simulink model "stopwatch_extended"  (Simulink 10.1)
settings: Solver=FixedStepAuto  StartTime=0.0  StopTime=1000.0  FixedStep=1e-3  RelTol=1e-3
settings Model: Creator=Robin Vogt  LastModifiedBy=Robin Vogt  EnablePacing=on
settings DataIOCC: SaveFormat=Dataset  ReturnWorkspaceOutputs=on
settings OptimizationCC: LifeSpan=auto
settings DebuggingCC: UnderspecifiedInitializationDetection=Simplified  MergeDetectMultiDrivingBlocksExec=error  SFUnexpectedBacktrackingDiag=error  SFNoUnconditionalDefaultTransitionDiag=error  SFExecutionAtInitializationDiag=warning  ArithmeticOperatorsInVariantConditions=error
settings HardwareCC: ProdBitPerPointer=64  ProdBitPerSizeT=64  ProdBitPerPtrDiffT=64  ProdLargestAtomicFloat=Float  ProdIntDivRoundTo=Zero  ProdEndianess=LittleEndian  ProdWordSize=64  ProdHWDeviceType=Intel->x86-64 (Windows64)
settings ModelReferenceCC: PropagateSignalLabelsOutOfModel=on
settings SFSimCC: SimUseLocalCustomCode=on  CustomCodeUndefinedFunction=FilterOut
settings RTWCC: RTWUseLocalCustomCode=on
settings CodeAppCC: StateflowObjectComments=off
settings GRTTargetCC: TargetLangStandard=C99 (ISO)  CombineOutputUpdateFcns=on  GRTInterface=off
settings ConfigComp: CovMetricSettings=dwe  CovHtmlReporting=off  CovSaveCumulativeToWorkspaceVar=off  CovSaveSingleToWorkspaceVar=off  CovExternalEMLEnable=on

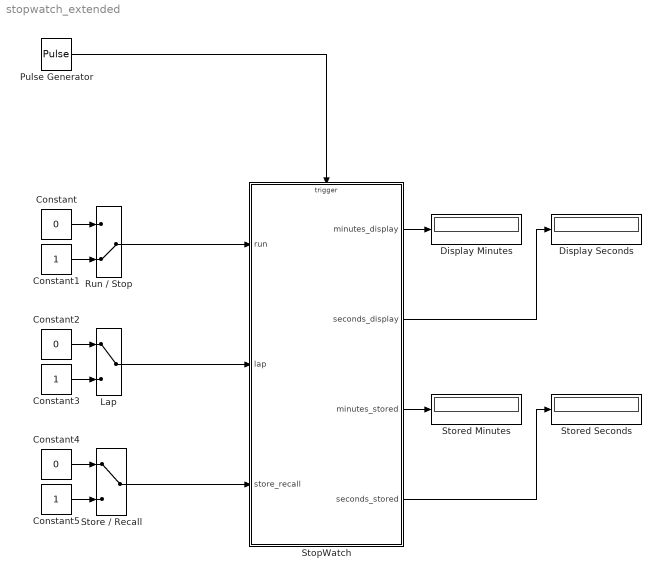
== system stopwatch_extended ==
  Constant : Constant  Value=0  OutDataTypeStr=boolean
  Constant1 : Constant  OutDataTypeStr=boolean
  Constant2 : Constant  Value=0  OutDataTypeStr=boolean
  Constant3 : Constant  OutDataTypeStr=boolean
  Constant4 : Constant  Value=0  OutDataTypeStr=boolean
  Constant5 : Constant  OutDataTypeStr=boolean
  Display Minutes : Display
  Display Seconds : Display
  Lap : ManualSwitch
  Pulse Generator : DiscretePulseGenerator  PulseType=Time based  Period=1  PulseWidth=5
  Run / Stop : ManualSwitch  CurrentSetting=0
  StopWatch : Stateflow chart  TreatAsAtomicUnit=on
  Store / Recall : ManualSwitch
  Stored Minutes : Display
  Stored Seconds : Display
  wires:
  Constant/1 -> Run / Stop/1
  Constant1/1 -> Run / Stop/2
  Run / Stop/1 -> StopWatch/1(run)
  Constant3/1 -> Lap/2
  Constant2/1 -> Lap/1
  StopWatch/2(seconds_display) -> Display Seconds/1
  StopWatch/1(minutes_display) -> Display Minutes/1
  Constant4/1 -> Store / Recall/1
  Constant5/1 -> Store / Recall/2
  Lap/1 -> StopWatch/2(lap)
  Pulse Generator/1 -> StopWatch/Trigger
  StopWatch/3(minutes_stored) -> Stored Minutes/1
  StopWatch/4(seconds_stored) -> Stored Seconds/1
  Store / Recall/1 -> StopWatch/3(store_recall)

== stateflow chart StopWatch ==
  settings: executeAtInitialization=1
  state Stopped
    state Reset
    state Paused
    state Paused_2
    (default) -> Paused
    Paused_2 -> Reset : [~store_recall]/
        | {
        | minutes = 0;
        | seconds = 0;
        | minutes_stored = 0;
        | seconds_stored = 0;
        | }
    Paused -> Paused_2 : [store_recall]/
        | {
        | minutes_stored = minutes;
        | seconds_stored = seconds;
        | }
  state Started
    state store_recall [parallel]
      settings: executionOrder=1
      state Recalled
      state Stored
      (default) -> Recalled
      Stored -> Recalled : [~store_recall]/
          | {
          | minutes = minutes_stored;
          | seconds = seconds_stored;
          | }
      Recalled -> Stored : [store_recall]/
          | {
          | minutes_stored = minutes;
          | seconds_stored = seconds;
          | }
    state Count [parallel]
      settings: executionOrder=2
      state Count
      (default) -> Started.Count.Count
      Started.Count.Count -> Started.Count.Count [order 1] : [seconds < 59]/
          | {
          | seconds = seconds +1;
          | }
      Started.Count.Count -> Started.Count.Count [order 2] : [seconds == 59]/
          | {
          | minutes = minutes +1;
          | seconds = 0;
          | }
    state Lap [parallel]
      settings: executionOrder=3
      state Lapped
      (default) -> Lapped
      Lapped -> Lapped : [~lap]/
          | {
          | minutes_display = minutes;
          | seconds_display = seconds;
          | }
  (default) -> Stopped
  Stopped -> Started : [run]
  Started -> Stopped : [~run]
  data: run input boolean; seconds local uint8 =uint8(0); minutes local uint32 =uint32(0); minutes_display output uint32; seconds_display output uint8; lap input boolean; minutes_stored output uint32; seconds_stored output uint8; store_recall input boolean
  events: clk input RISING_EDGE_EVENT
